simulink model "linearsim_slx"  (R2022a)
settings: Solver=ode15s  StartTime=0.0  StopTime=simset.stop_time  FixedStep=simset.sampletime  MaxStep=simset.max_step_size  RelTol=1e-3
values from neighbouring files (symbols this model uses):
  dydx = struct2vec(response, y_fds)    [shape_cinv_controlsim.m]
  sys = models{i}    [close_vs_loops.m]    (also in estimate_radial_gains.m = response_models([], tok, 0, 0, 'vacuum'); estimate_vertical_gains.m = sys{1}; response_models.m = struct; rzip_analysis.m)
  x0 = [eq.ic; eq.iv; eq.cpasma]    [shape_cinv_controlsim.m]
  y0 = struct2vec(y0data, y_fds)    [shape_cinv_controlsim.m]    (also in vs_hinfstruct.m = [])
undefined symbols (not defined in the file or in its folder): PS
libraries: cstblocks x1
settings Model: Creator=jwai  LastModifiedBy=jwai

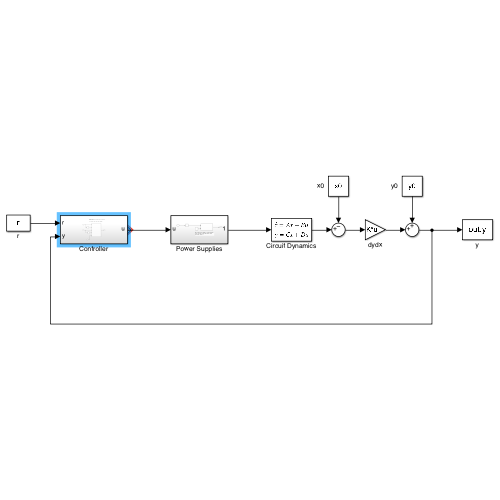
[thumbnail: Simulink's stored preview of the top-level diagram]
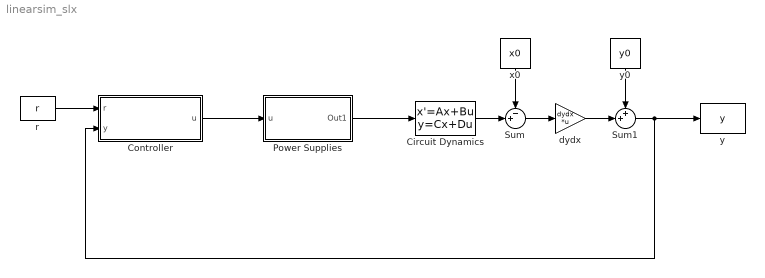
== system linearsim_slx ==
  Circuit Dynamics : StateSpace  A=sys.amat  B=sys.bmat  C=eye(size(sys.amat))  D=zeros(size(sys.bmat))  InitialCondition=0
  Controller : Subsystem
  Power Supplies : Subsystem
  Sum : Sum  Inputs=-+|
  Sum1 : Sum  Inputs=++|
  dydx : Gain  Gain=dydx  Multiplication=Matrix(K*u)
  r : FromWorkspace  VariableName=r
  x0 : Constant  Value=x0
  y : ToWorkspace  VariableName=y  SaveFormat=Timeseries  SampleTime=-1
  y0 : Constant  Value=y0
  wires:
  Circuit Dynamics/1 -> Sum/2
  Sum/1 -> dydx/1
  dydx/1 -> Sum1/2
  x0/1 -> Sum/1
  y0/1 -> Sum1/1
  r/1 -> Controller/1(r)
  Power Supplies/1(Out1) -> Circuit Dynamics/1
  Sum1/1 -> Controller/2(y), y/1
  Controller/1(u) -> Power Supplies/1(u)

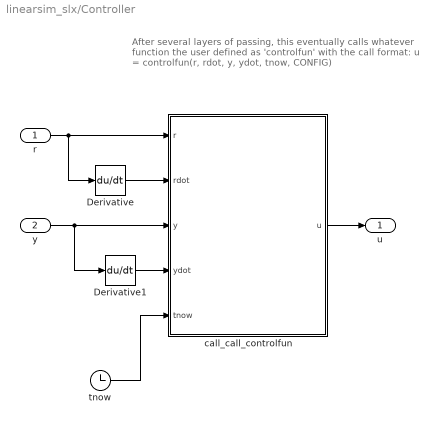
== system linearsim_slx/Controller ==
  note: After several layers of passing, this eventually calls
      | whatever function the user defined as 'controlfun' with
      | the call format:
      |
      | u = controlfun(r, rdot, y, ydot, tnow, CONFIG)
  r : Inport
  y : Inport  Port=2
  Derivative : Derivative  CoefficientInTFapproximation=1e-6
  Derivative1 : Derivative
  call_call_controlfun : MATLAB Function  TreatAsAtomicUnit=on
  tnow : Clock
  u : Outport
  wires:
  r/1 -> Derivative/1, call_call_controlfun/1(r)
  call_call_controlfun/1(u) -> u/1
  Derivative1/1 -> call_call_controlfun/4(ydot)
  tnow/1 -> call_call_controlfun/5(tnow)
  Derivative/1 -> call_call_controlfun/2(rdot)
  y/1 -> Derivative1/1, call_call_controlfun/3(y)

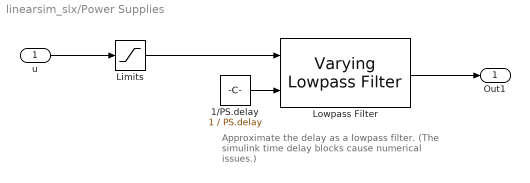
== system linearsim_slx/Power Supplies ==
  note: Approximate the delay as a lowpass filter.
      | (The simulink time delay blocks cause
      | numerical issues.)
  u : Inport
  1/PS.delay : Constant  Value=1 / PS.delay
  Limits : Saturate  UpperLimit=PS.vmax  LowerLimit=PS.vmin
  Lowpass Filter : cstblocks/Linear Parameter Varying/Varying Lowpass Filter  N=1
  Out1 : Outport
  wires:
  u/1 -> Limits/1
  Lowpass Filter/1 -> Out1/1
  Limits/1 -> Lowpass Filter/1
  1/PS.delay/1 -> Lowpass Filter/2

== matlab function linearsim_slx/Controller/call_call_controlfun ==
  data: r input; rdot input; u output; y input size=[circ.nc,1]; ydot input; tnow input; CONFIG parameter
function u = call_call_controlfun(r, rdot, y, ydot, tnow, CONFIG)

coder.extrinsic('call_controlfun')
u = zeros(8,1);
u = call_controlfun(r, rdot, y, ydot, tnow, CONFIG);
